simulink model "Final_Model_Project2_TaskB"  (R2023b)
settings: Solver=ode4  StartTime=0.0  StopTime=1.0  FixedStep=2e-6  RelTol=1e-3
values from neighbouring files (symbols this model uses):
  f_g = 50    [Project2.m]
  f_s = 50    [Project2.m]
  J = 1200    [Project2.m]
  L_lr = 0.06492e-03    (= 6.492e-05)    [Project2.m]
  L_ls = 0.06492e-03    (= 6.492e-05)    [Project2.m]
  P = 2    [Project2.m]
  R_r = 1.497e-03    (= 0.001497)    [Project2.m]
  R_s = 1.102e-03    (= 0.001102)    [Project2.m]
  S_sR = 2.59e06    (= 2590000)    [Project2.m]
  slip = (n_syn - n_minit)/n_syn    (= 0.0333333333333)    [Project2.m]
  V_gLL = 690    [Project2.m]
  V_sLL = 690    [Project2.m]
libraries: spsAsynchronousMachineSIUnitsLib x1, spsGroundLib x1, spsThreePhaseProgrammableVoltageSourceLib x1, sps_lib x1
settings Model: Creator=priya  LastModifiedBy=priya
settings SolverCC: AutoInsertRateTranBlk=on

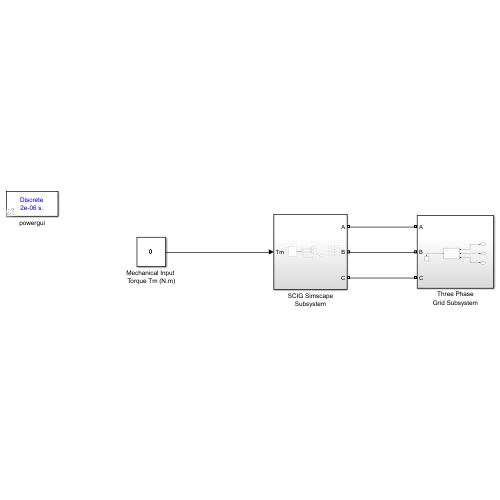
[thumbnail: Simulink's stored preview of the top-level diagram]
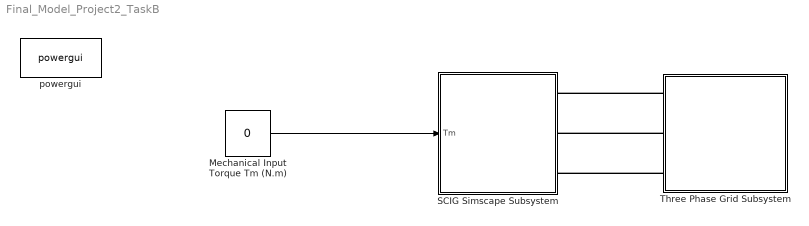
== system Final_Model_Project2_TaskB ==
  Mechanical Input Torque Tm (N.m) : Constant  Value=0
  SCIG Simscape Subsystem : Subsystem
  Three Phase Grid Subsystem : Subsystem
  powergui : sps_lib/powergui  Priority=1  SimulationMode=Discrete  SampleTime=2e-06  frequency=60  Iterations=50  frequencyindice=50  Pbase=100e6  ErrMax=1e-4  UnitsV=kV  UnitsW=MW  buscounter=0  FunctionMessages=off  echomessages=off  EnableUseOfTLC=off  CurrentSourceSwitches=off  DisableSnubberDevices=off  DisableRonSwitches=off  DisableVfSwitches=off  DisplayEquations=off  AutomaticDiscreteSolvers=off  SolverType=Tustin/Backward Euler (TBE)  Interpol=off  ExternalGateDelay=off  methode=off  Ts=100  x0status=blocks  SPID=on  SwTol=0  HookPort=off  NonlinearTolerance=1e-4  nMaxIteration=100  ContinueOnMaxIteration=off  RestoreLinks=warning  ResistiveCurrentMeasurement=off  Frange=[0:2:500]  Ylog=off  Xlog=on  ShowGrid=off  save=off  variable=ZData  structure=0  ZoomFFT=off  StartTime=0.0  cycles=1  DisplayStyle=1  fundamental=60  FreqAxis=off  MaxFrequency=1000  frequencyindicesteady=1  RmsSteady=1  display=off
  wires:
  Mechanical Input Torque Tm (N.m)/1 -> SCIG Simscape Subsystem/1(Tm)
  connections:
  Three Phase Grid Subsystem/LConn1 -- SCIG Simscape Subsystem/RConn1
  Three Phase Grid Subsystem/LConn2 -- SCIG Simscape Subsystem/RConn2
  Three Phase Grid Subsystem/LConn3 -- SCIG Simscape Subsystem/RConn3

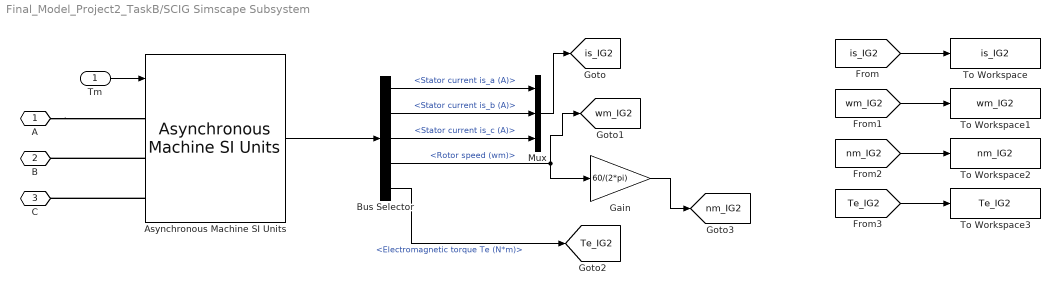
== system Final_Model_Project2_TaskB/SCIG Simscape Subsystem ==
  Tm : Inport
  Asynchronous Machine SI Units : spsAsynchronousMachineSIUnitsLib/Asynchronous Machine SI Units  RotorType=Squirrel-cage  PresetModel=No  MechanicalLoad=Torque Tm  ShowDetailedParameters=on  ReferenceFrame=Stationary  Units=SI  MeasurementBus=off  NominalParameters=[S_sR V_sLL f_s]  VoltageRatio=1  Stator=[R_s L_ls]  Rotor=[R_r L_lr]  Cage1=[0.4155 0.002066]  Cage2=[0.4168 0.0003495]  Lm=L_m  Mechanical=[J 0 P]  PolePairs=2  InitialConditions=[slip 0 0 0 0 0 0 0]  SimulateSaturation=off  Saturation=[14.03593122, 27.81365428, 53.79336849, 72.68890987, 97.98006896, 148.6815601, 215.7428561, 302.9841135, 428.7778367 ; 230, 322, 414, 460, 506, 552, 598, 644, 690]  LoadFlowParameters=1492000  TsPowergui=0  TsBlock=-1  IterativeModel=Trapezoidal non iterative  IterativeDiscreteModel=Trapezoidal non iterative  Pmec=1.492e+006
  Bus Selector : BusSelector  OutputSignals=Stator measurements.Stator current is_a (A),Stator measurements.Stator current is_b (A),Stator measurements.Stator current is_c (A),Mechanical.Rotor speed (wm),Mechanical.Electromagnetic torque Te (N*m)
  Gain : Gain  Gain=60/(2*pi)
  Mux : Mux  Inputs=3
  To Workspace : ToWorkspace  VariableName=is_IG2  SampleTime=-1
  To Workspace1 : ToWorkspace  VariableName=wm_IG2  SampleTime=-1
  To Workspace2 : ToWorkspace  VariableName=nm_IG2  SampleTime=-1
  To Workspace3 : ToWorkspace  VariableName=Te_IG2  SampleTime=-1
  A : PMIOPort  Side=Right
  B : PMIOPort  Port=2  Side=Right
  C : PMIOPort  Port=3  Side=Right
  tag scope: Te_IG2=global, is_IG2=global, nm_IG2=global, wm_IG2=global
  wires:
  Bus Selector/1 -> Mux/1  "<Stator current is_a (A)>"
  [wm_IG2] -> To Workspace1/1
  Gain/1 -> [nm_IG2]
  [Te_IG2] -> To Workspace3/1
  Bus Selector/3 -> Mux/3  "<Stator current is_c (A)>"
  Mux/1 -> [is_IG2]
  Bus Selector/4 -> [wm_IG2], Gain/1  "<Rotor speed (wm)>"
  [is_IG2] -> To Workspace/1
  [nm_IG2] -> To Workspace2/1
  Bus Selector/5 -> [Te_IG2]  "<Electromagnetic torque Te (N*m)>"
  Bus Selector/2 -> Mux/2  "<Stator current is_b (A)>"
  Asynchronous Machine SI Units/1 -> Bus Selector/1
  Tm/1 -> Asynchronous Machine SI Units/1
  connections:
  A/RConn1 -- Asynchronous Machine SI Units/LConn1
  Asynchronous Machine SI Units/LConn2 -- B/RConn1
  Asynchronous Machine SI Units/LConn3 -- C/RConn1

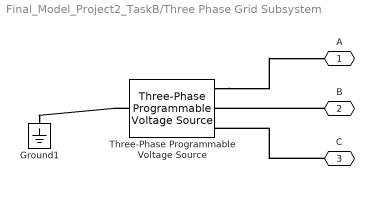
== system Final_Model_Project2_TaskB/Three Phase Grid Subsystem ==
  Ground1 : spsGroundLib/Ground  LConnTagsString=a
  Three-Phase Programmable Voltage Source : spsThreePhaseProgrammableVoltageSourceLib/Three-Phase Programmable Voltage Source  PositiveSequence="[V_gLL  0 f_g]"  VariationEntity=None  VariationType=Table of time-amplitude pairs  VariationTypeAlt=Step  VariationStep=0.5  VariationRate=10  VariationMagnitude=0.3  VariationFrequency=2  VariationTiming=[1 2]  VariationPhaseA=off  Amplitudes=[1 0.8 1.2 1.0]  TimeValues=[0 0.1 0.15 0.2]  HarmonicGeneration=off  HarmonicA=[3 0.2 -25 0]  HarmonicB=[2 0.15 35 2]  Timing="[0.05  3]"  BusType=swing  Pref=0  Qref=0  Qmin=-inf  Qmax=inf
  A : PMIOPort  Side=Left
  B : PMIOPort  Port=2  Side=Left
  C : PMIOPort  Port=3  Side=Left
  connections:
  Three-Phase Programmable Voltage Source/LConn1 -- Ground1/LConn1
  B/RConn1 -- Three-Phase Programmable Voltage Source/RConn2
  C/RConn1 -- Three-Phase Programmable Voltage Source/RConn3
  Three-Phase Programmable Voltage Source/RConn1 -- A/RConn1
